simulink model "nncACCsystem"  (R2018a)
settings: Solver=FixedStepAuto  StartTime=0.0  StopTime=T  RelTol=1e-3
values from neighbouring files (symbols this model uses):
  seed = randi([0,1000])    [generateOnetrace.m]
  t_gap = 1.4    [generateOnetrace.m]
  Ts = 0.1    [generateOnetrace.m]
  v0_ego = 20 + 1.5 - 3*rand(1)    [generateOnetrace.m]
  v0_lead = 25 + 1.5 - 3*rand(1)    [generateOnetrace.m]
  v_set = 30    [generateOnetrace.m]
  x0_ego = 10 + 1.5 - 3*rand(1)    [generateOnetrace.m]
  x0_lead = 50 + 1.5 - 3*rand(1)    [generateOnetrace.m]
libraries: neural x35
(part 2 of 2)

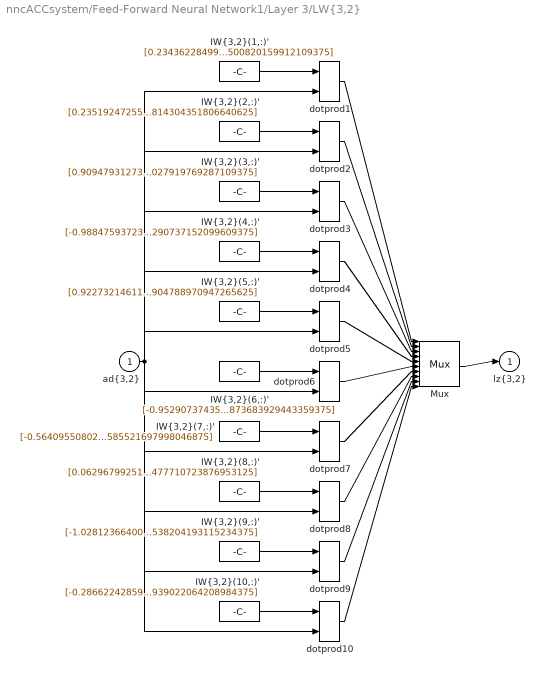
== system nncACCsystem/Feed-Forward Neural Network1/Layer 3/LW{3,2} ==
  "ad{3,2}" : Inport  PortDimensions=10
      mask Display: e = 0.06;c1 = [120 230 180]/255;c2 = ([120 230 180]+0)/(256+128);c3 = ([120 230 180]+128)/(256+128);patch([0 1 1 0],[0 0 1 1],c1);patch([0 1 1 1-e 1-e 0+e],[0 0 1 1-e 0+e 0+e],c2);patch([0 0 1 1-e 0+e 0+e],[0 1 1 1-e 1-e 0+e],c3);plot([0 1 1 0 0],[0 0 1 1 0]);
  "IW{3,2}(1,:)'" : Constant  Value=[0.2343622849966617849304384435527026653289794921875;0.781941122877345407005122979171574115753173828125;0.1677123552110157955752356429002247750759124755859375;-0.0851187996256239642889340757392346858978271484375;-0.621203282376784127194468965171836316585540771484375;-0.8060771786764444613027080777101218700408935546875;0.214802207170997849772220433806069195270538330078125;-0.1772025292445997823875813992344774305820465087890625;-0.8109923858873162583194016406196169555187225341796875;0.4506139734193046475496657876647077500820159912109375]
      mask Display: e = 0.06;c1 = [120 150 230]/255;c2 = ([120 150 230]+0)/383;c3 = ([120 150 230]+128)/383;patch([0 1 1 0],[0 0 1 1],c1);patch([0 1 1 1-e 1-e 0+e],[0 0 1 1-e 0+e 0+e],c2);patch([0 0 1 1-e 0+e 0+e],[0 1 1 1-e 1-e 0+e],c3);plot([0 1 1 0 0],[0 0 1 1 0]);disp('weights');
  "IW{3,2}(10,:)'" : Constant  Value=[-0.286622428590477207333009346257313154637813568115234375;-0.592868293606418905739019464817829430103302001953125;-0.2026677247083963351315105683170258998870849609375;0.090489173125406441311469052379834465682506561279296875;-0.67565107245176403427677769286674447357654571533203125;0.41609243313621580018235590614494867622852325439453125;0.62643858733603929866973203388624824583530426025390625;-0.0394378756076901593186079253428033553063869476318359375;-0.9112554715672589455977004035958088934421539306640625;-0.492886103764980931796202412442653439939022064208984375]
      mask Display: e = 0.06;c1 = [120 150 230]/255;c2 = ([120 150 230]+0)/383;c3 = ([120 150 230]+128)/383;patch([0 1 1 0],[0 0 1 1],c1);patch([0 1 1 1-e 1-e 0+e],[0 0 1 1-e 0+e 0+e],c2);patch([0 0 1 1-e 0+e 0+e],[0 1 1 1-e 1-e 0+e],c3);plot([0 1 1 0 0],[0 0 1 1 0]);disp('weights');
  "IW{3,2}(2,:)'" : Constant  Value=[0.235192472551532472113677840752643533051013946533203125;0.43964633276222375712904977262951433658599853515625;0.9154514240173179384640889111324213445186614990234375;-0.0203520185936119681058276142948670894838869571685791015625;-0.436958634039496474077424181814421899616718292236328125;0.32402888746401925512685693320236168801784515380859375;0.280327102041962594736190794719732366502285003662109375;0.7153204449771644046762730795308016240596771240234375;0.9538358837252918220883657340891659259796142578125;0.53697749652451565172128766789683140814304351806640625]
      mask Display: e = 0.06;c1 = [120 150 230]/255;c2 = ([120 150 230]+0)/383;c3 = ([120 150 230]+128)/383;patch([0 1 1 0],[0 0 1 1],c1);patch([0 1 1 1-e 1-e 0+e],[0 0 1 1-e 0+e 0+e],c2);patch([0 0 1 1-e 0+e 0+e],[0 1 1 1-e 1-e 0+e],c3);plot([0 1 1 0 0],[0 0 1 1 0]);disp('weights');
  "IW{3,2}(3,:)'" : Constant  Value=[0.9094793127399671828214877677964977920055389404296875;-0.2026390215731590505043868688517250120639801025390625;-0.429045524354080998197247254211106337606906890869140625;-0.26729729828373838262933759324369020760059356689453125;-0.628163729440098794754021582775749266147613525390625;0.6745449903162905602727050791145302355289459228515625;-0.7877051667735226470057341430219821631908416748046875;-0.13643957661691807903281414837692864239215850830078125;-0.260066850721384523748014316879562102258205413818359375;0.004667216181276544195721811547628021799027919769287109375]
      mask Display: e = 0.06;c1 = [120 150 230]/255;c2 = ([120 150 230]+0)/383;c3 = ([120 150 230]+128)/383;patch([0 1 1 0],[0 0 1 1],c1);patch([0 1 1 1-e 1-e 0+e],[0 0 1 1-e 0+e 0+e],c2);patch([0 0 1 1-e 0+e 0+e],[0 1 1 1-e 1-e 0+e],c3);plot([0 1 1 0 0],[0 0 1 1 0]);disp('weights');
  "IW{3,2}(4,:)'" : Constant  Value=[-0.9884759372398093102418670241604559123516082763671875;-0.9189863730948284459287833669804967939853668212890625;-0.379478083010867328628279437907622195780277252197265625;0.60616143031091496151674391512642614543437957763671875;0.9249259578518438384975297594792209565639495849609375;-0.477049489548897032165086784516461193561553955078125;-0.7928462933021969138991380532388575375080108642578125;0.848737509664243550133733151596970856189727783203125;-0.062338898740715943669332688159556710161268711090087890625;-0.352712581415149661889785193125135265290737152099609375]
      mask Display: e = 0.06;c1 = [120 150 230]/255;c2 = ([120 150 230]+0)/383;c3 = ([120 150 230]+128)/383;patch([0 1 1 0],[0 0 1 1],c1);patch([0 1 1 1-e 1-e 0+e],[0 0 1 1-e 0+e 0+e],c2);patch([0 0 1 1-e 0+e 0+e],[0 1 1 1-e 1-e 0+e],c3);plot([0 1 1 0 0],[0 0 1 1 0]);disp('weights');
  "IW{3,2}(5,:)'" : Constant  Value=[0.9227321461156778870105199530371464788913726806640625;0.949353829860247966365704996860586106777191162109375;0.90890498455852852810465947186457924544811248779296875;-0.2494266172320342700441386796228471212089061737060546875;0.99751132354809712854404324389179237186908721923828125;0.309535527202363935916906712009222246706485748291015625;-0.6876507490927308285932895159930922091007232666015625;-0.77672483290959204449421804383746348321437835693359375;-0.845968211161998606684164769831113517284393310546875;-0.03275858630317508846108154330067918635904788970947265625]
      mask Display: e = 0.06;c1 = [120 150 230]/255;c2 = ([120 150 230]+0)/383;c3 = ([120 150 230]+128)/383;patch([0 1 1 0],[0 0 1 1],c1);patch([0 1 1 1-e 1-e 0+e],[0 0 1 1-e 0+e 0+e],c2);patch([0 0 1 1-e 0+e 0+e],[0 1 1 1-e 1-e 0+e],c3);plot([0 1 1 0 0],[0 0 1 1 0]);disp('weights');
  "IW{3,2}(6,:)'" : Constant  Value=[-0.952907374350325131473482542787678539752960205078125;0.36905394345097786157339214696548879146575927734375;0.11709550243656684231918774230507551692426204681396484375;-0.323652348692822500186849765668739564716815948486328125;0.058217621643134258302421102371226879768073558807373046875;-0.06055956446471046084045752877500490285456180572509765625;0.077387403655915676381482626311480998992919921875;0.7242171758939071057881164961145259439945220947265625;0.30400132065985119300677297360380180180072784423828125;-1.212678710836966100572453797212801873683929443359375]
      mask Display: e = 0.06;c1 = [120 150 230]/255;c2 = ([120 150 230]+0)/383;c3 = ([120 150 230]+128)/383;patch([0 1 1 0],[0 0 1 1],c1);patch([0 1 1 1-e 1-e 0+e],[0 0 1 1-e 0+e 0+e],c2);patch([0 0 1 1-e 0+e 0+e],[0 1 1 1-e 1-e 0+e],c3);plot([0 1 1 0 0],[0 0 1 1 0]);disp('weights');
  "IW{3,2}(7,:)'" : Constant  Value=[-0.56409550802349739395680217057815752923488616943359375;-0.1109988177960075095285219504148699343204498291015625;-0.0490389057201242317685085936318500898778438568115234375;0.232273757524974922006322231027297675609588623046875;0.2906861780851739407438572015962563455104827880859375;-1.1100129827151870021140211974852718412876129150390625;-0.2327479321708662285406177261393168009817600250244140625;0.50374393366776326619316250798874534666538238525390625;-0.07566913425665643122552950217141187749803066253662109375;-0.101381695374666402909014095712336711585521697998046875]
      mask Display: e = 0.06;c1 = [120 150 230]/255;c2 = ([120 150 230]+0)/383;c3 = ([120 150 230]+128)/383;patch([0 1 1 0],[0 0 1 1],c1);patch([0 1 1 1-e 1-e 0+e],[0 0 1 1-e 0+e 0+e],c2);patch([0 0 1 1-e 0+e 0+e],[0 1 1 1-e 1-e 0+e],c3);plot([0 1 1 0 0],[0 0 1 1 0]);disp('weights');
  "IW{3,2}(8,:)'" : Constant  Value=[0.0629679925189974287746963454992510378360748291015625;0.624201896389141364096531106042675673961639404296875;0.646644405819616796549098580726422369480133056640625;-0.3054406377916978332365260939695872366428375244140625;0.1832065592006102416888779771397821605205535888671875;-0.1726226494684570678117552233743481338024139404296875;-0.602691106634114959206272033043205738067626953125;-0.3440645123486394396650212001986801624298095703125;-0.478626533144882682080378799582831561565399169921875;-0.3588725871403941614090626899269409477710723876953125]
      mask Display: e = 0.06;c1 = [120 150 230]/255;c2 = ([120 150 230]+0)/383;c3 = ([120 150 230]+128)/383;patch([0 1 1 0],[0 0 1 1],c1);patch([0 1 1 1-e 1-e 0+e],[0 0 1 1-e 0+e 0+e],c2);patch([0 0 1 1-e 0+e 0+e],[0 1 1 1-e 1-e 0+e],c3);plot([0 1 1 0 0],[0 0 1 1 0]);disp('weights');
  "IW{3,2}(9,:)'" : Constant  Value=[-1.0281236640004574045548224603408016264438629150390625;0.8209742894285010361699050918105058372020721435546875;0.791548527048598682398505843593738973140716552734375;0.85766259884193141171948582268669269979000091552734375;0.278994300725670274498924072759109549224376678466796875;-0.288048795406173729904963920489535667002201080322265625;0.025417162540666775327746762513925204984843730926513671875;-0.5076263388829669320756465822341851890087127685546875;0.95743447223318811634129588128416799008846282958984375;0.553366009055176188979885409935377538204193115234375]
      mask Display: e = 0.06;c1 = [120 150 230]/255;c2 = ([120 150 230]+0)/383;c3 = ([120 150 230]+128)/383;patch([0 1 1 0],[0 0 1 1],c1);patch([0 1 1 1-e 1-e 0+e],[0 0 1 1-e 0+e 0+e],c2);patch([0 0 1 1-e 0+e 0+e],[0 1 1 1-e 1-e 0+e],c3);plot([0 1 1 0 0],[0 0 1 1 0]);disp('weights');
  Mux : Mux  Inputs=10
      mask Display: e = 0.06;c1 = [120 150 230]/255;c2 = ([120 150 230]+0)/383;c3 = ([120 150 230]+128)/383;patch([0 1 1 0],[0 0 1 1],c1);patch([0 1 1 1-e 1-e 0+e],[0 0 1 1-e 0+e 0+e],c2);patch([0 0 1 1-e 0+e 0+e],[0 1 1 1-e 1-e 0+e],c3);plot([0 1 1 0 0],[0 0 1 1 0]);disp('Mux');
  dotprod{1..10} (10 alike) : neural/Weight Functions/dotprod
  "lz{3,2}" : Outport
      mask Display: e = 0.06;c1 = [120 230 180]/255;c2 = ([120 230 180]+0)/(256+128);c3 = ([120 230 180]+128)/(256+128);patch([0 1 1 0],[0 0 1 1],c1);patch([0 1 1 1-e 1-e 0+e],[0 0 1 1-e 0+e 0+e],c2);patch([0 0 1 1-e 0+e 0+e],[0 1 1 1-e 1-e 0+e],c3);plot([0 1 1 0 0],[0 0 1 1 0]);
  wires:
  "IW{3,2}(1,:)'"/1 -> dotprod1/1
  "ad{3,2}"/1 -> dotprod1/2, dotprod2/2, dotprod3/2, dotprod4/2, dotprod5/2, dotprod6/2, dotprod7/2, dotprod8/2, dotprod9/2, dotprod10/2
  dotprod1/1 -> Mux/1
  "IW{3,2}(2,:)'"/1 -> dotprod2/1
  dotprod2/1 -> Mux/2
  "IW{3,2}(3,:)'"/1 -> dotprod3/1
  dotprod3/1 -> Mux/3
  "IW{3,2}(4,:)'"/1 -> dotprod4/1
  dotprod4/1 -> Mux/4
  "IW{3,2}(5,:)'"/1 -> dotprod5/1
  dotprod5/1 -> Mux/5
  "IW{3,2}(6,:)'"/1 -> dotprod6/1
  dotprod6/1 -> Mux/6
  "IW{3,2}(7,:)'"/1 -> dotprod7/1
  dotprod7/1 -> Mux/7
  "IW{3,2}(8,:)'"/1 -> dotprod8/1
  dotprod8/1 -> Mux/8
  "IW{3,2}(9,:)'"/1 -> dotprod9/1
  dotprod9/1 -> Mux/9
  "IW{3,2}(10,:)'"/1 -> dotprod10/1
  dotprod10/1 -> Mux/10
  Mux/1 -> "lz{3,2}"/1

== system nncACCsystem/Feed-Forward Neural Network1/Layer 4/Delays 1 ==
  "p{4}" : Inport  PortDimensions=10
      mask Display: e = 0.06;c1 = [120 230 180]/255;c2 = ([120 230 180]+0)/(256+128);c3 = ([120 230 180]+128)/(256+128);patch([0 1 1 0],[0 0 1 1],c1);patch([0 1 1 1-e 1-e 0+e],[0 0 1 1-e 0+e 0+e],c2);patch([0 0 1 1-e 0+e 0+e],[0 1 1 1-e 1-e 0+e],c3);plot([0 1 1 0 0],[0 0 1 1 0]);
  mux : Mux  Inputs=1
      mask Display: e = 0.06;c1 = [120 150 230]/255;c2 = ([120 150 230]+0)/383;c3 = ([120 150 230]+128)/383;patch([0 1 1 0],[0 0 1 1],c1);patch([0 1 1 1-e 1-e 0+e],[0 0 1 1-e 0+e 0+e],c2);patch([0 0 1 1-e 0+e 0+e],[0 1 1 1-e 1-e 0+e],c3);plot([0 1 1 0 0],[0 0 1 1 0]);disp('Mux')
  "pd{4,3}" : Outport
      mask Display: e = 0.06;c1 = [120 230 180]/255;c2 = ([120 230 180]+0)/(256+128);c3 = ([120 230 180]+128)/(256+128);patch([0 1 1 0],[0 0 1 1],c1);patch([0 1 1 1-e 1-e 0+e],[0 0 1 1-e 0+e 0+e],c2);patch([0 0 1 1-e 0+e 0+e],[0 1 1 1-e 1-e 0+e],c3);plot([0 1 1 0 0],[0 0 1 1 0]);
  wires:
  "p{4}"/1 -> mux/1
  mux/1 -> "pd{4,3}"/1

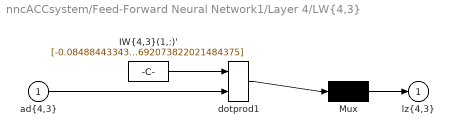
== system nncACCsystem/Feed-Forward Neural Network1/Layer 4/LW{4,3} ==
  "ad{4,3}" : Inport  PortDimensions=10
      mask Display: e = 0.06;c1 = [120 230 180]/255;c2 = ([120 230 180]+0)/(256+128);c3 = ([120 230 180]+128)/(256+128);patch([0 1 1 0],[0 0 1 1],c1);patch([0 1 1 1-e 1-e 0+e],[0 0 1 1-e 0+e 0+e],c2);patch([0 0 1 1-e 0+e 0+e],[0 1 1 1-e 1-e 0+e],c3);plot([0 1 1 0 0],[0 0 1 1 0]);
  "IW{4,3}(1,:)'" : Constant  Value=[-0.0848844334301210867721465547219850122928619384765625;-0.0117681277778264488376169794037195970304310321807861328125;-0.0842085066493206968463169914684840478003025054931640625;-0.71893932798435200570708047962398268282413482666015625;0.0232320077732809486537046694820674019865691661834716796875;0.215583913460868636935430231460486538708209991455078125;1.3586855731060742957794218455092050135135650634765625;0.982971401872842154290310645592398941516876220703125;-0.01406817082182458718275785969353819382376968860626220703125;0.14424868925502509764413616721867583692073822021484375]
      mask Display: e = 0.06;c1 = [120 150 230]/255;c2 = ([120 150 230]+0)/383;c3 = ([120 150 230]+128)/383;patch([0 1 1 0],[0 0 1 1],c1);patch([0 1 1 1-e 1-e 0+e],[0 0 1 1-e 0+e 0+e],c2);patch([0 0 1 1-e 0+e 0+e],[0 1 1 1-e 1-e 0+e],c3);plot([0 1 1 0 0],[0 0 1 1 0]);disp('weights');
  Mux : Mux  Inputs=1
      mask Display: e = 0.06;c1 = [120 150 230]/255;c2 = ([120 150 230]+0)/383;c3 = ([120 150 230]+128)/383;patch([0 1 1 0],[0 0 1 1],c1);patch([0 1 1 1-e 1-e 0+e],[0 0 1 1-e 0+e 0+e],c2);patch([0 0 1 1-e 0+e 0+e],[0 1 1 1-e 1-e 0+e],c3);plot([0 1 1 0 0],[0 0 1 1 0]);disp('Mux');
  dotprod1 : neural/Weight Functions/dotprod
  "lz{4,3}" : Outport
      mask Display: e = 0.06;c1 = [120 230 180]/255;c2 = ([120 230 180]+0)/(256+128);c3 = ([120 230 180]+128)/(256+128);patch([0 1 1 0],[0 0 1 1],c1);patch([0 1 1 1-e 1-e 0+e],[0 0 1 1-e 0+e 0+e],c2);patch([0 0 1 1-e 0+e 0+e],[0 1 1 1-e 1-e 0+e],c3);plot([0 1 1 0 0],[0 0 1 1 0]);
  wires:
  "IW{4,3}(1,:)'"/1 -> dotprod1/1
  "ad{4,3}"/1 -> dotprod1/2
  dotprod1/1 -> Mux/1
  Mux/1 -> "lz{4,3}"/1
